simulink model "Sweep Generater"  (R2026a)
settings: Solver=FixedStepAuto  StopTime=80  FixedStep=0.01
settings Model: Creator=Jay  LastModifiedBy=Jay

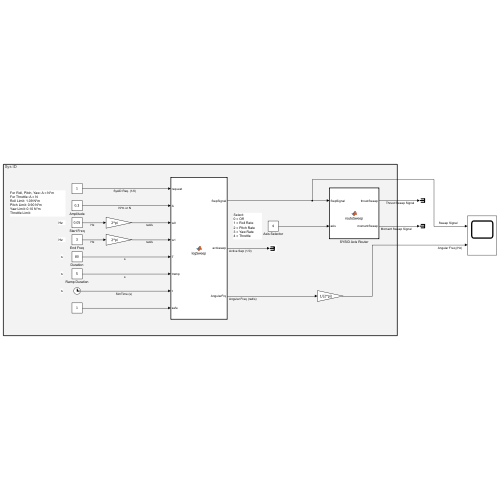
[thumbnail: Simulink's stored preview of the top-level diagram]
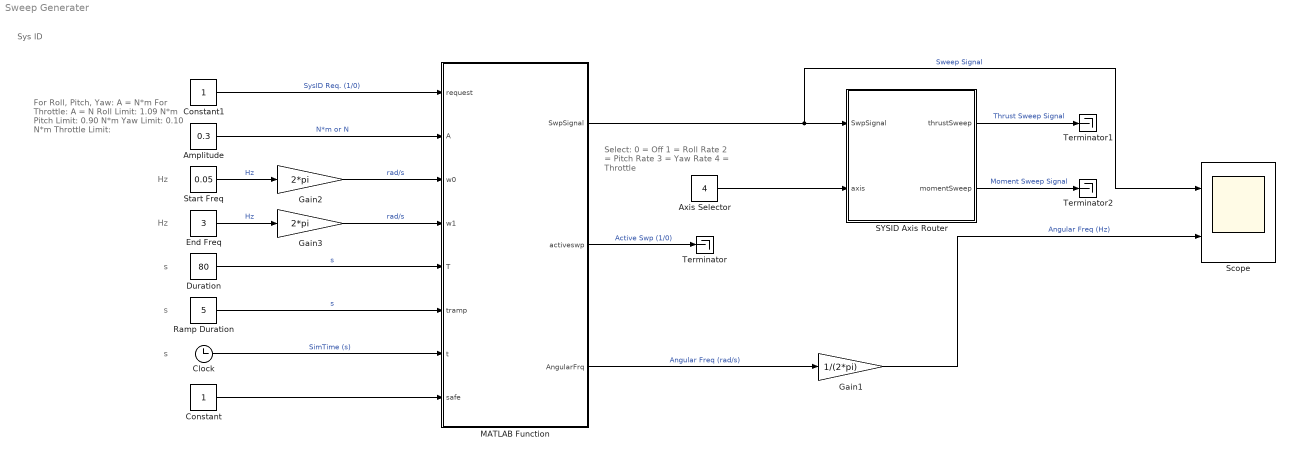
== system Sweep Generater ==
  note: For Roll, Pitch, Yaw: A = N*m
      | For Throttle: A = N
      | Roll Limit: 1.09 N*m
      | Pitch Limit: 0.90 N*m
      | Yaw Limit: 0.10 N*m
      | Throttle Limit:
  note: Sys ID
  note: s
  note: s
  note: Hz
  note: s
  note: Select:
      | 0 = Off
      | 1 = Roll Rate
      | 2 = Pitch Rate
      | 3 = Yaw Rate
      | 4 = Throttle
  note: Hz
  Amplitude : Constant  Value=0.3
  Axis Selector : Constant  Value=4
  Clock : Clock
  Constant : Constant
  Constant1 : Constant
  Duration : Constant  Value=80
  End Freq : Constant  Value=3
  Gain1 : Gain  Gain=1/(2*pi)
  Gain2 : Gain  Gain=2*pi
  Gain3 : Gain  Gain=2*pi
  MATLAB Function : MATLAB Function  TreatAsAtomicUnit=on
  Ramp Duration : Constant  Value=5
  SYSID Axis Router : MATLAB Function  TreatAsAtomicUnit=on
  Scope : Scope  NumInputPorts=2
      settings: ActiveDisplayYMinimum=-0.62500000000000022  ActiveDisplayYMaximum=5.6250000000000027
  Start Freq : Constant  Value=0.05
  Terminator : Terminator
  Terminator1 : Terminator
  Terminator2 : Terminator
  wires:
  MATLAB Function/3(AngularFrq) -> Gain1/1  "Angular Freq (rad/s)"
  Gain2/1 -> MATLAB Function/3(w0)  "rad/s"
  Duration/1 -> MATLAB Function/5(T)  "s"
  MATLAB Function/2(activeswp) -> Terminator/1  "Active Swp (1/0)"
  Clock/1 -> MATLAB Function/7(t)  "SimTime (s)"
  MATLAB Function/1(SwpSignal) -> Scope/1, SYSID Axis Router/1(SwpSignal)  "Sweep Signal"
  Gain3/1 -> MATLAB Function/4(w1)  "rad/s"
  Amplitude/1 -> MATLAB Function/2(A)  "N*m or N"
  Ramp Duration/1 -> MATLAB Function/6(tramp)  "s"
  SYSID Axis Router/1(thrustSweep) -> Terminator1/1  "Thrust Sweep Signal"
  Constant1/1 -> MATLAB Function/1(request)  "SysID Req. (1/0)"
  End Freq/1 -> Gain3/1  "Hz"
  SYSID Axis Router/2(momentSweep) -> Terminator2/1  "Moment Sweep Signal"
  Start Freq/1 -> Gain2/1  "Hz"
  Axis Selector/1 -> SYSID Axis Router/2(axis)
  Constant/1 -> MATLAB Function/8(safe)
  Gain1/1 -> Scope/2  "Angular Freq (Hz)"

== matlab function Sweep Generater/SYSID Axis Router ==
  data: thrustSweep output; momentSweep output; SwpSignal input; axis input
function [thrustSweep, momentSweep] = routeSweep(SwpSignal,axis)
%#codegen

momentSweep = [0.0 0.0 0.0];
thrustSweep = 0.0;

if axis == 1
    momentSweep(1) = SwpSignal;      % roll moment
elseif axis == 2
    momentSweep(2) = SwpSignal;      % pitch moment
elseif axis == 3
    momentSweep(3) = SwpSignal;      % yaw moment
elseif axis == 4
    thrustSweep = SwpSignal;         % collective thrust
end

== matlab function Sweep Generater/MATLAB Function ==
  settings: updateMethod=DISCRETE
  data: SwpSignal output; request input; A input; w0 input; w1 input; T input; tramp input; activeswp output; AngularFrq output; t input; safe input
function [SwpSignal,activeswp,AngularFrq] = logSweep( ...
    request,A,w0,w1,T,tramp,t,safe)

%% Keeps Memory of variables so that the function doesn't forget the
%  maneuver is began so that it isn't beginning every time step again
persistent tStart previousRequest aborted

if isempty(tStart)
    tStart = 0.0;
    previousRequest = false;
    aborted = false;
end

SwpSignal = 0.0;  activeswp = 0.0;  AngularFrq = 0.0; % Default Outputs and True/False statements

enabled = request > 0.5;  safeNow = safe > 0.5; % 1/0 or True/False

%% Turning the request off rearms the generator.
if ~enabled
    previousRequest = false;
    aborted = false;
    return
end

%% Any unsafe condition aborts the maneuver.
if ~safeNow
    previousRequest = true;
    aborted = true;
    return
end

%% Start only on a new request and assign start time of Sweep
if ~previousRequest
    tStart = t;
end

previousRequest = true;

%% An aborted maneuver cannot resume until request is toggled off.
if aborted
    return
end

% Tau is start of freq. swp. not t which is start of simulation
tau = t - tStart; % s

%%  When swp. time is finished, only starts a new swp. when controller
 %  switch is cycled off and back on
valid = tau >= 0.0 && tau <= T && ... 
    T > 0.0 && w0 > 0.0 && w1 > 0.0;  % True/False

%% Sweep Generation
% For Roll, Pitch, Yaw axis: A = N/m and for Throttle: A = N
if valid
    beta = log(w1/w0)/T; % Hz (1/s)

    if abs(beta) < 1.0e-9
        AngularFrq = w0; % Hz (1/s)
        phase = w0*tau;  % rads
    else
        exponentialTerm = exp(beta*tau);
        AngularFrq = w0*exponentialTerm;           % Hz (1/s)
        phase = (w0/beta)*(exponentialTerm - 1.0); % rads
    end

%% Finds time where Ramp is active at beginning and end of Sweep and
%  creates envelope which is a fade in and fade out 
ramp = max(0.0,min(tramp,T/2.0)); % s
envelope = 1.0;

    if ramp > 0.0
        if tau < ramp
            envelope = 0.5*(1.0-cos(pi*tau/ramp));
        elseif tau > T-ramp
            envelope = 0.5*(1.0-cos(pi*(T-tau)/ramp));
        end
    end

%% Actual swp. signal
    SwpSignal = A*envelope*sin(phase);
    activeswp = 1.0;
end
